simulink model "block_diagram"  (R2023a)
settings: Solver=VariableStepAuto  StartTime=0.0  StopTime=10.0  RelTol=1e-3
values from neighbouring files (symbols this model uses):
  A = A_prime_ave / (b * constat_V_to_m_ave)    [main_code.m]
  b = ending_step_value_ave - start_step_value_ave    [main_code.m]    (also in simulation - Copy.m = 1)
undefined symbols (not defined in the file or in its folder): C, K
settings Model: Creator=kianf  LastModifiedBy=kianf

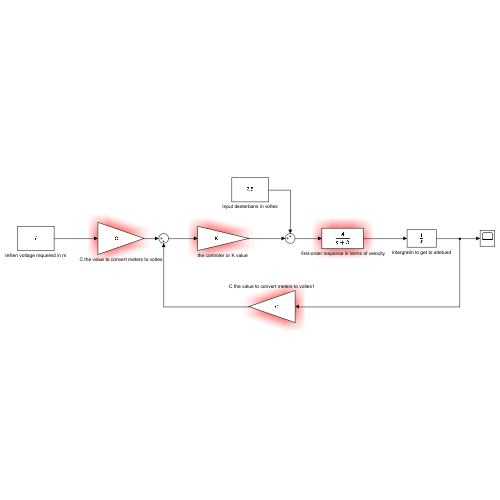
[thumbnail: Simulink's stored preview of the top-level diagram]
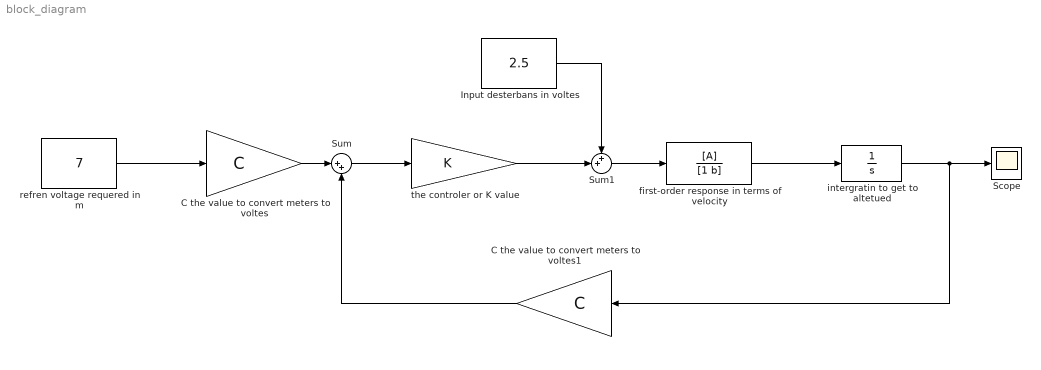
== system block_diagram ==
  " first-order response in terms of velocity" : TransferFcn  Numerator=[A]  Denominator=[1 b]
  C the value to convert meters to voltes : Gain  Gain=C
  C the value to convert meters to voltes1 : Gain  Gain=C
  Input desterbans in voltes : Constant  Value=2.5
  Scope : Scope
  Sum : Sum  Inputs=|++
  Sum1 : Sum  Inputs=++|
  intergratin to get to altetued : TransferFcn  Denominator=[1 0]
  refren voltage requered in m : Constant  Value=7
  "the controler or K value " : Gain  Gain=K
  wires:
  refren voltage requered in m/1 -> C the value to convert meters to voltes/1
  C the value to convert meters to voltes/1 -> Sum/1
  Sum/1 -> "the controler or K value "/1
  "the controler or K value "/1 -> Sum1/2
  Input desterbans in voltes/1 -> Sum1/1
  Sum1/1 -> " first-order response in terms of velocity"/1
  " first-order response in terms of velocity"/1 -> intergratin to get to altetued/1
  intergratin to get to altetued/1 -> Scope/1, C the value to convert meters to voltes1/1
  C the value to convert meters to voltes1/1 -> Sum/2
